simulink model "ex1a"  (R2015a)
settings: Solver=ode45  StartTime=0.0  StopTime=10.0  RelTol=1e-3
settings Model: Creator=ayush  LastModifiedBy=ayush

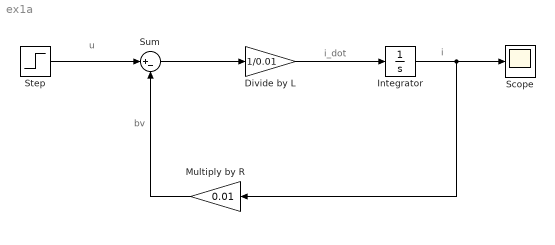
== system ex1a ==
  note: bv
  note: i
  note: i_dot
  note: u
  Divide by L : Gain  Gain=1/0.01
  Integrator : Integrator
  Multiply by R : Gain  Gain=0.01
  Scope : Scope
  Step : Step  Time=0  After=400  SampleTime=0
  Sum : Sum  Inputs=|+-
  wires:
  Sum/1 -> Divide by L/1
  Divide by L/1 -> Integrator/1
  Integrator/1 -> Multiply by R/1, Scope/1
  Step/1 -> Sum/1
  Multiply by R/1 -> Sum/2
